simulink model "sysmecanique"  (R2024a)
settings: Solver=VariableStepAuto  StartTime=0.0  StopTime=30  RelTol=1e-3
model workspace (MAT data in the model file):
  K = 2
undefined symbols (not defined in the file): b, M
settings Model: Creator=hp  LastModifiedBy=NB
settings SolverCC: AlgebraicLoopSolver=TrustRegion
settings DataIOCC: ReturnWorkspaceOutputs=off
settings DebuggingCC: UnconnectedInputMsg=warning  UnconnectedOutputMsg=warning  UnconnectedLineMsg=warning  ArithmeticOperatorsInVariantConditions=warning
settings ModelReferenceCC: EnableRefExpFcnMdlSchedulingChecks=on
settings SFSimCC: CustomCodeUndefinedFunction=UseInterfaceOnly
settings RTWCC: GPUComputeCapability=3.5

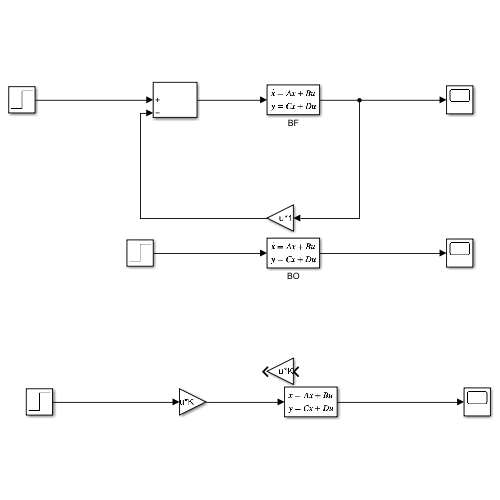
[thumbnail: Simulink's stored preview of the top-level diagram]
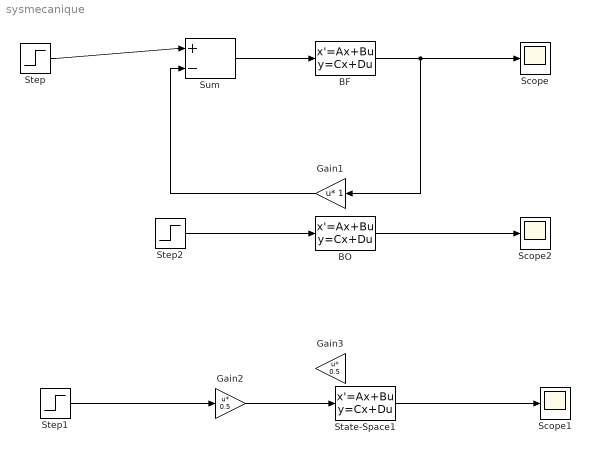
== system sysmecanique ==
  BF : StateSpace  A=[0,1;-0.666666666666667,-2.666666666666667]  B=[0;0.333333333333333]  C=[1 0]  D=0  InitialCondition=0
  BO : StateSpace  A=[0,1;-0.666666666666667,-2.666666666666667]  B=[0;0.333333333333333]  C=[1 0]  D=0  InitialCondition=0
  Gain1 : Gain  Multiplication=Matrix(u*K)
  Gain2 : Gain  Gain=0.5  Multiplication=Matrix(u*K)
  Gain3 : Gain  Gain=0.5  Multiplication=Matrix(u*K)
  Scope : Scope
  Scope1 : Scope
  Scope2 : Scope
  State-Space1 : StateSpace  A=[0 1;-K/M -b/M]  B=[0;1/M]  C=[1 0]  D=0  InitialCondition=0
  Step : Step  Time=0  SampleTime=0
  Step1 : Step  SampleTime=0
  Step2 : Step  Time=0  SampleTime=0
  Sum : Sum  Inputs=|+-
  wires:
  Sum/1 -> BF/1
  BF/1 -> Gain1/1, Scope/1
  Gain1/1 -> Sum/2
  Gain2/1 -> State-Space1/1
  State-Space1/1 -> Scope1/1
  Step1/1 -> Gain2/1
  Step/1 -> Sum/1
  BO/1 -> Scope2/1
  Step2/1 -> BO/1
